simulink library "PowerFlowLib"  (Simulink 8.1)
settings: Solver=ode45  StartTime=0.0  StopTime=10.0  RelTol=1e-3
undefined symbols (not defined in the file or in its folder): AirProp, C, F1, Fanmap, Fld1, Fld2, Fluid, fueltankdata, HydProp, HydraulicLoad, IBFD_exc, L, LoadFluidProps, magnitude, MSSN, n_alghts, PumpProp, pwr_alghts, R_fd_exc, Rcore, Ts, VBFD_exc
libraries: PowerFlowLib x33, simulink x15, powerlib_extras x2, dspstat3 x2
(part 6 of 11)

== system PowerFlowLib/Energy & Power Systems/Thermal/Fuel & Oil ==
  Cold Plate : Subsystem  mask{fld=Fuel, Tw_init=50, C_wall=60000, H0=10000, A=0.033217, mdot0=2, Q0=12750, Tw0=50, Tin0=10}
      mask prompts: fld "Fluid Type"; Tw_init "Initial Wall Temperature [°C]"; C_wall "Wall Heat Capacitance [J/K]"; H0 "Heat Transfer Coefficient [W/m²K]"; A "Heat Transfer Area [m²]"; mdot0 "Mass Flow Rate [kg/s]"; Q0 "Heat Absorption Rate [W]"; Tw0 "Wall Temperature [°C]"; Tin0 "Fluid Inlet Temperature [°C]"
      mask init:
      | load Fluids
      | eval(['Fluid = Fluid.',get_param(gcb,'fld'),';']);
      | 
      | 
      | area = -(mdot0*Fluid.cp/H0)*...
      |               log(1-Q0/(mdot0*Fluid.cp*(Tw0-Tin0)));
      |           
      |           
      | set_param(gcb,'A',num2str(area));
      mask TypeOptions fld: Fuel | Water
      mask Display:
      | text(0.5,0.95,['{\bf ',fld,' Cold Plate}'],'TexMode','on','horizontalAlignment', 'center')
      | 
      | port_label('input',1,'Heat Load [W]')
      | port_label('input',2,'Flow In')
      | port_label('output',1,'Flow Out')
  Flow Junction : Subsystem  Description=TwoPhase  mask{fld=Fuel, V=.05, Bm=10^5, initPres=6000, initTemp=30}
      mask prompts: fld "Fluid Type"; V "Volume (m^3)"; Bm "Bulk Modulus (kPa)"; initPres "Initial Pressure (kPa)"; initTemp "Initial Temperature (C)"
      mask init:
      | initTemp = initTemp + 273.15;
      | if strcmp(get_param(gcb,'fld'),'Fuel') == 1
      |     load FluidProp_JetA3638
      |     eval(['F1 = FuelProp;']);
      | elseif strcmp(get_param(gcb,'fld'),'Oil') == 1
      |     load OilProp
      |     eval(['F1 = OilProp;']);
      | else
      |     error(['Incorrect fluid chosen in block: ',gcb,'.  Check initialization commands.'])
      | end
      mask TypeOptions fld: Fuel | Oil
      mask Display:
      | image(imread('MergeImage.png'))
      | 
      | port_label('input',1,'{\bf mdot Out}','TexMode','on')
      | port_label('input',2,'{\bf Flow 1}','TexMode','on')
      | port_label('input',3,'{\bf Flow 2}','TexMode','on')
      | port_label('input',4,'{\bf Flow 3}','TexMode','on')
      | 
      | port_label('output',1,'{\bfFlow }','TexMode','on')
  Fluid Pump : Subsystem  mask(Pump){fld=Fuel, maptype=Pressure (kPa) vs. Vol. Flow Rate (m³/hr), map=B737_mech_fuel1, map_load=off, SG=0.82, pump_eff=.75, heat_out=on, AC_pwr=on, pf=1, mech_pwr=off}
      mask prompts: fld "Fluid Type"; maptype "Map Type"; map "Select Map"; map_load "Load new map?"; SG "Specific Gravity of Flow"; pump_eff "Pump Overall Efficiency"; heat_out "Add heat to flow?"; AC_pwr "AC Powered?"; pf "Power Factor"; mech_pwr "Mechanically Driven?"
      mask help:
      | Input 1: Input Flow Bus
      | Input 2: Shaft RPM (rpm)
      | Input 3: Upstream Pressure (kPa)
      |
      | Output 1: Output Flow Bus
      | Output 2: Pump Power Bus (mech or elec)
      | Optional: Pump Heat Generated (kW)
      mask init:
      | if exist('PumpProp') == 0
      |   load('PumpProp.mat')
      | end
      | h      = get_param(gcb,'handle');   % Get block handle
      | blk    = gcb; 
      | hblock = get(h);     % Parse out handles structure
      | 
      | if strcmp(get_param(gcb,'fld'),'Fuel') == 1
      |     load FluidProp_JetA3638
      |     eval(['F1 = FuelProp;']);
      | elseif strcmp(get_param(gcb,'fld'),'Oil') == 1
      |     load OilProp
      |     eval(['F1 = OilProp;']);
      | else
      |     error(['Incorrect fluid chosen in block: ',gcb,'.  Check initialization commands.'])
      | end
      | 
      | if strcmp(hblock.maptype,'Head (m) vs. Vol. Flow Rate (m³/hr)') == 1;
      |     set_param([blk,'/switchcase'],'Value','1');
      |     set_param([blk,'/Pump Vol. FlowRate'],'Table',['PumpProp.',map,'.q']);
      |     set_param([blk,'/Pump Vol. FlowRate'],'BreakpointsForDimension1',['PumpProp.',map,'.head']);
      | elseif strcmp(hblock.maptype,'Pressure (kPa) vs. Vol. Flow Rate (m³/hr)') == 1;
      |     set_param([blk,'/switchcase'],'Value','2');
      |     set_param([blk,'/Pump Vol. FlowRate'],'Table',['PumpProp.',map,'.q']);
      |     set_param([blk,'/Pump Vol. FlowRate'],'BreakpointsForDimension1',['PumpProp.',map,'.pres']);
      | elseif strcmp(hblock.maptype,'Pressure (bar) vs. Vol. Flow Rate (m³/hr)') == 1;
      |     set_param([blk,'/switchcase'],'Value','3');
      |     set_param([blk,'/Pump Vol. FlowRate'],'Table',['PumpProp.',map,'.q']);
      |     set_param([blk,'/Pump Vol. FlowRate'],'BreakpointsForDimension1',['PumpProp.',map,'.pres']);
      | else
      |     error('see pump mask callback for map type');
      | end    
      | 
      | % TURNING ON/OFF PUMP HEAT GENERATION OUTPUT
      | if strcmp(hblock.heat_out,'on') == 1;   % adding heat to fluid flow
      |     set_param([blk,'/heat_switch'],'Gain','1')  % turn on heat added to flow
      |     try
      |         delete_block([blk,'/Heat (kW)'])
      |     catch
      |     end
      |     delete_unconnected_lines(blk)
      |         
      | elseif strcmp(hblock.heat_out,'off') == 1; % not adding heat to fluid flow
      |     set_param([blk,'/heat_switch'],'Gain','0')  % adding no heat to flow
      |     try
      |         add_block('built-in/Outport',[blk,'/Heat (kW)'],'Position',[800 200 830 214]);
      |         add_line(blk,'W to kW/1','Heat (kW)/1')
      |     catch
      |     end
      | end
      | 
      | clear h blk hblock
      settings: OpenFcn=|
      | if exist('PumpProp') == 0
      |   load('PumpProp.mat')
      | end
      | open_system(gcb,'mask')
      mask TypeOptions fld: Fuel | Oil
      mask TypeOptions maptype: Head (m) vs. Vol. Flow Rate (m³/hr) | Pressure (kPa) vs. Vol. Flow Rate (m³/hr) | Pressure (bar) vs. Vol. Flow Rate (m³/hr)
      mask Callback maptype:
      | h      = get_param(gcb,'handle');   % Get block handle
      | blk    = gcb;
      | hblock = get(h);     % Parse out handles structure
      | 
      | if strcmp(hblock.maptype,'Head (m) vs. Vol. Flow Rate (m³/hr)') == 1;
      |     set_param([blk,'/switchcase'],'Value','1');
      |     set_param([blk,'/Pump Vol. FlowRate'],'Table',['PumpProp.',hblock.map,'.q']);
      |     set_param([blk,'/Pump Vol. FlowRate'],'BreakpointsForDimension1',['PumpProp.',hblock.map,'.head']);
      | elseif strcmp(hblock.maptype,'Pressure (kPa) vs. Vol. Flow Rate (m³/hr)') == 1;
      |     set_param([blk,'/switchcase'],'Value','2');
      |     set_param([blk,'/Pump Vol. FlowRate'],'Table',['PumpProp.',hblock.map,'.q']);
      |     set_param([blk,'/Pump Vol. FlowRate'],'BreakpointsForDimension1',['PumpProp.',hblock.map,'.pres']);
      | elseif strcmp(hblock.maptype,'Pressure (bar) vs. Vol. Flow Rate (m³/hr)') == 1;
      |     set_param([blk,'/switchcase'],'Value','3');
      |     set_param([blk,'/Pump Vol. FlowRate'],'Table',['PumpProp.',hblock.map,'.q']);
      |     set_param([blk,'/Pump Vol. FlowRate'],'BreakpointsForDimension1',['PumpProp.',hblock.map,'.pres']);
      | else
      |     error('see pump mask callback for map type');
      | end
      | 
      | clear h blk hblock
      mask TypeOptions map: B737_mech_fuel1 | B737_mech_fuel2 | B737_mech_fuel3 | B737_AC_fuel1 | B737_AC_oil1
      mask Callback map:
      | h      = get_param(gcb,'handle');   % Get block handle
      | blk    = gcb;
      | hblock = get(h);     % Parse out handles structure
      | vals = get_param(blk,'MaskValues');
      | % find all installed pumps in the PumpProp.mat file
      | pumps = fieldnames(PumpProp);
      | indx = strfind(pumps, 'units');
      | indx = find(not(cellfun('isempty', indx)));
      | pumps(indx) = [];      % removing the units entry
      | 
      | for i = 1:size(pumps,1);
      |    if i==1;
      |     pmpstr = pumps{i};
      |    else
      |        pmpstr = strcat(pmpstr,char(124),pumps{i});
      |    end
      | end
      | 
      | % Get the mask parameter values. This is a cell array of strings.
      | styl = get_param(blk,'MaskStyles');
      | 
      | vis = get_param(blk,'MaskVisibilities');
      | str = get_param(blk,'MaskPromptString');
      | 
      | % fill the mask with the parameters
      | set_param(blk,'MaskVisibilities',vis,'MaskPromptString',str,'MaskValues',vals,'MaskStyles',[styl(1:2);strcat('popup(',pmpstr,')');styl(4:10)]);
      | 
      | clear h blk hblock styl vals vis str pmpstr i indx pumps
      mask Callback AC_pwr:
      | h      = get_param(gcb,'handle');   % Get block handle
      | blk    = gcb;
      | hblock = get(h);     % Parse out handles structure
      | 
      | vis = get_param(blk,'MaskVisibilities');
      | 
      | if strcmp(hblock.AC_pwr,'off') == 1;
      |     % fill the mask with the parameters
      |     set_param(blk,'MaskVisibilities',[vis(1:8);'off';vis(10)])
      |     set_param(blk,'mech_pwr','on');
      |     set_param([blk,'/pwr_switch'],'Value','0.5')
      | elseif strcmp(hblock.AC_pwr,'on') == 1;
      |     % fill the mask with the parameters
      |     set_param(blk,'MaskVisibilities',[vis(1:8);'on';vis(10)])
      |     set_param(blk,'mech_pwr','off');
      |     set_param([blk,'/pwr_switch'],'Value','0')
      | end
      | 
      | clear h blk hblock vis
      mask Callback mech_pwr:
      | h      = get_param(gcb,'handle');   % Get block handle
      | blk    = gcb;
      | hblock = get(h);     % Parse out handles structure
      | 
      | vis = get_param(blk,'MaskVisibilities');
      | 
      | if strcmp(hblock.mech_pwr,'off') == 1;
      |     % fill the mask with the parameters
      |     set_param(blk,'MaskVisibilities',[vis(1:8);'on';vis(10)])
      |     set_param(blk,'AC_pwr','on');
      |     set_param([blk,'/pwr_switch'],'Value','0')
      | elseif strcmp(hblock.mech_pwr,'on') == 1;
      |     % fill the mask with the parameters
      |     set_param(blk,'MaskVisibilities',[vis(1:8);'off';vis(10)])
      |     set_param(blk,'AC_pwr','off');
      |     set_param([blk,'/pwr_switch'],'Value','0.5')
      | end
      | clear h blk hblock vis
      mask Display:
      | image(imread('pump.png'));
      | 
      | port_label('input',1,'{\bf Flow In}','TexMode','on')
      | port_label('input',2,'{\bf w (rpm)}','TexMode','on')
      | port_label('input',3,'{\bf P_o_u_t (kPa)}','TexMode','on')
      | 
      | port_label('output',1,'{\bf Flow Out}','TexMode','on')
      | port_label('output',2,'{\bf Pump Power}','TexMode','on')
      | 
      | h      = get_param(gcb,'handle');   % Get block handle
      | hblock = get(h);     % Parse out handles structure
      | 
      | if heat_out == 0
      |     port_label('output',3,'{\bf Pump Heat [kW]}','TexMode','on')
      | end
  Fluid Tank : Subsystem  mask(Fluid Tank){fld=Fuel, fileslct=off, filename=fueltank_area.m, filedir=fueltank_area.m, tank_loc=Left Wing Tank, areaprompt2=off, max_vol=3.2, m_init=2500, fld_Tint=0, ull_Tint=30, Pover=100, HTC_fg=14.2, wallHXF=off, wetHTC=14.2, dryHTC=14.2, Qinternal=0}
      mask prompts: fld "Fluid Type"; fileslct "Browse for area .m file?"; filename "Fuel Tank Area .m File"; filedir "Area .m File Directory"; tank_loc "Select Tank"; areaprompt2 "Edit Fuel Tank Area Manually?"; max_vol "Maximum Tank Volume [m³]"; m_init "Initial Fluid Mass [kg]"; fld_Tint "Initial Fluid Temperature [°C]"; ull_Tint "Initial Ullage Temperature [°C]"; Pover "Tank Pressurization [kPa]"; HTC_fg "Liquid to Ullage HTC [W/m² K]"; wallHXF "Enable Wall Heat Transfer"; wetHTC "Wall to Liquid HTC [W/m² K]"; dryHTC "Wall to Ullage HTC [W/m² K]"; Qinternal "Internal Heat Load [W]"
      mask help:
      | Input 1: Input Flow Bus
      | Input 2: Flow Rate Out [kg/s]
      | Input 3: Ambient Pressure [kPa]
      | Input 4: Heat Load [W]
      | Input 5: Initial Wall Temps. Vector [K]
      |
      | Output 1: Output Flow Bus
      | Output 2: Tank mass [kg]
      | Output 3: Ullage Temp. [K]
      mask init:
      | h      = get_param(gcb,'handle');   % Get block handle
      | blk    = gcb; 
      | hblock = get(h);     % Parse out handles structure 
      | 
      | if strcmp(get_param(gcb,'fld'),'Fuel') == 1
      |     load FluidProp_JetA3638
      |     eval(['F1 = FuelProp;']);
      | elseif strcmp(get_param(gcb,'fld'),'Oil') == 1
      |     load OilProp
      |     eval(['F1 = OilProp;']);
      | else
      |     error(['Incorrect fluid chosen in block: ',gcb,'.  Check initialization commands.'])
      | end
      | 
      | if exist('AirProp') == 0
      |     load AirProp.mat
      | end
      | %{
      | % the following checks for the existance of a file and loads the
      | % spreadsheet into variables that populate the 2D lookup table
      | 
      | if isempty(filedir) == 0;
      |     areadata = xlsread(filedir,1);
      |     vol_per = areadata(:,1);
      |     wall_area = [areadata(:,2:size(areadata,2))];
      | end
      | %}
      | if strcmp(hblock.areaprompt2,'on') == 0;
      |     
      |     % run the selected fuel area file
      |     if ~isempty(strfind(filename,'.m'))
      |         try
      |             run(filename(1:strfind(filename,'.m')-1))       % removing the .m extension and loading the file
      |         catch
      |             error(['Unable to load selected fuel area file in ',blk,'. Verify the file is a .m script file and on the MATLAB Path'])
      |         end
      |     else
      |         try
      |             run(filename)
      |         catch
      |             error(['Unable to load selected fuel area file in ',blk,'. Verify the file is a .m script file and on the MATLAB Path'])
      |         end
      |     end
      |    
      |     switch hblock.tank_loc
      |         case 'Left Wing Tank'
      |             set_param([blk,'/Wall Heat Transfer/volume_%'],'Table', 'fueltankdata.leftwingtank');
      |             %BP1values = strcat('[',num2str(linspace(0,1,size(fueltankdata.leftwingtank,1))),']');
      |             %BP2values = strcat('[',num2str(linspace(1,size(fueltankdata.leftwingtank,2),size(fueltankdata.leftwingtank,2))),']');
      |             set_param([blk,'/Wall Heat Transfer/volume_%'],'BreakpointsForDimension1', 'linspace(0,1,11)');
      |             set_param([blk,'/Wall Heat Transfer/volume_%'],'BreakpointsForDimension2', 'linspace(1,6,6)');
      |             set_param([blk,'/Wall Heat Transfer/Walls 1 to n'],'Value','1:size(fueltankdata.leftwingtank,2)');
      |             set_param([blk,'/Wall Heat Transfer/total area'],'Bias','-[fueltankdata.leftwingtank(11,:)]');
      |             set_param([blk,'/ullage-fluid_area'],'Value','fueltankdata.leftwingtank(2,2)');
      |             
      |         case 'Center Tank'
      |             set_param([blk,'/Wall Heat Transfer/volume_%'],'Table', 'fueltankdata.centertank');
      |             %BP1values = strcat('[',num2str(linspace(0,1,size(fueltankdata.centertank,1))),']');
      |             %BP2values = strcat('[',num2str(linspace(1,size(fueltankdata.centertank,2),size(fueltankdata.centertank,2))),']');
      |             set_param([blk,'/Wall Heat Transfer/volume_%'],'BreakpointsForDimension1', 'linspace(0,1,11)');
      |             set_param([blk,'/Wall Heat Transfer/volume_%'],'BreakpointsForDimension2', 'linspace(1,6,6)');
      |             set_param([blk,'/Wall Heat Transfer/Walls 1 to n'],'Value','1:size(fueltankdata.centertank,2)');
      |             set_param([blk,'/Wall Heat Transfer/total area'],'Bias','-[fueltankdata.centertank(11,:)]');
      |             set_param([blk,'/ullage-fluid_area'],'Value','fueltankdata.centertank(2,2)');
      |             
      |         case 'Right Wing Tank'
      |             set_param([blk,'/Wall Heat Transfer/volume_%'],'Table', 'fueltankdata.rightwingtank');
      |             %BP1values = strcat('[',num2str(linspace(0,1,size(fueltankdata.rightwingtank,1))),']');
      |             %BP2values = strcat('[',num2str(linspace(1,size(fueltankdata.rightwingtank,2),size(fueltankdata.rightwingtank,2))),']');
      |             set_param([blk,'/Wall Heat Transfer/volume_%'],'BreakpointsForDimension1', 'linspace(0,1,11)');
      |             set_param([blk,'/Wall Heat Transfer/volume_%'],'BreakpointsForDimension2', 'linspace(1,6,6)');
      |             set_param([blk,'/Wall Heat Transfer/Walls 1 to n'],'Value','1:size(fueltankdata.rightwingtank,2)');
      |             set_param([blk,'/Wall Heat Transfer/total area'],'Bias','-[fueltankdata.rightwingtank(11,:)]');
      |             set_param([blk,'/ullage-fluid_area'],'Value','fueltankdata.rightwingtank(2,2)');
      |             
      |     end
      |     
      | end
      | 
      | %% CHECK FOR VOLUME OF FUEL BEING GREATER THAN VOLUME OF TANK
      | X = F1.P;
      | Y = F1.T;
      | delx = X(2)-X(1);
      | dely = Y(2)-Y(1);
      | xref = round((Pover + 101 - X(1))/delx);
      | yref = round((fld_Tint + 273 - Y(1))/dely);
      | 
      | rhoIC = F1.Rho_pt(xref,yref);
      | volIC = m_init / rhoIC;
      | 
      | if volIC > max_vol
      |     error('Initial volume of fluid is greater than max volume of tank.')
      | end
      | 
      | 
      | clear h blk hblock
      mask TypeOptions fld: Fuel | Oil
      mask Callback fileslct:
      | h      = get_param(gcb,'handle');   % Get block handle
      | blk    = gcb;
      | hblock = get(h);     % Parse out handles structure
      | 
      | if strcmp(hblock.fileslct,'on') == 1;
      |     set_param(gcb,'areaprompt2','off');     % turn off manual switch
      |     RR_SetPerfSlct(2,0);                    % call uiopen script
      |     set_param(gcb,'fileslct','off')
      | end
      | 
      | clear h blk hblock
      mask TypeOptions tank_loc: Left Wing Tank | Center Tank | Right Wing Tank
      mask Callback areaprompt2:
      | h      = get_param(gcb,'handle');   % Get block handle
      | blk    = gcb;
      | hblock = get(h);     % Parse out handles structure
      | 
      | if strcmp(hblock.areaprompt2,'on') == 1;
      |     set_param(gcb,'fileslct','off');
      |     open_system([blk, '/Wall Heat Transfer/volume_%']);
      | end
      mask Callback wallHXF:
      | h      = get_param(gcb,'handle');   % Get block handle
      | blk    = gcb;
      | hblock = get(h);     % Parse out handles structure
      | 
      | if strcmp(hblock.wallHXF,'on') == 1;
      |     set_param([blk,'/enable_wall_HXF'],'Value','1');
      | else
      |     set_param([blk,'/enable_wall_HXF'],'Value','0');
      | end
      | 
      | clear h blk hblock
      mask Display:
      | image(imread('fueltank.jpg'))
      | 
      | port_label('input',1,'{\bf Flow In}','TexMode','on')
      | port_label('input',2,'{\bf Flow Rate Out}','TexMode','on')
      | port_label('input',3,'{\bf P_a_m_b [kPa]}','TexMode','on')
      | port_label('input',4,'{\bf Heat Load [kW]}','TexMode','on')
      | port_label('input',5,'{\bf Wall Temp. [K]}','TexMode','on')
      | 
      | port_label('output',1,'{\bf Flow Out }','TexMode','on')
      | port_label('output',2,'{\bf Fluid Mass [kg]}','TexMode','on')
      | port_label('output',3,'{\bf Ullage Temp. [K]}','TexMode','on')
  Fuel Control : Subsystem  mask(Fuel Control){}
      mask help: Manages fuel bypass and fuel sent to the engine.
      mask Display:
      | port_label('input',1,'{\bf Fuel Need}','TexMode','on')
      | port_label('input',2,'{\bf Fuel In}','TexMode','on')
      | 
      | 
      | port_label('output',1,'{\bf Fuel to Eng.}','TexMode','on')
      | port_label('output',2,'{\bf Fuel Return}','TexMode','on')
  Heat Exchanger : Subsystem  mask(Single-phase Fluid Heat Exchanger){fld1=Fuel, fld2=Air, Tw_init=0, C_wall=60000, Tw0=30, Q0=20000, H1_0=10000, A1=0.11584, mdot1_0=2, Tin1_0=10, Pin1_0=100, H2_0=10000, A2=0.13814, mdot2_0=2, Tin2_0=50, Pin2_0=100}
      mask prompts: fld1 "Fluid Type 1"; fld2 "Fluid Type 2"; Tw_init "Initial Wall Temperature [°C]"; C_wall "Wall Heat Capacitance  [J/K]"; Tw0 "Wall Temperature [°C]"; Q0 "Heat Transfer Rate [W]"; H1_0 "Heat Transfer Coefficient [W/m²K]"; A1 "Heat Transfer Area [m²]"; mdot1_0 "Mass Flow Rate [kg/s]"; Tin1_0 "Fluid Inlet Temperature [°C]"; Pin1_0 "Fluid Inlet Pressure [kPa]"; H2_0 "Heat Transfer Coefficient [W/m²K]"; A2 "Heat Transfer Area [m²]"; mdot2_0 "Mass Flow Rate [kg/s]"; Tin2_0 "Fluid Inlet Temperature [°C]"; Pin2_0 "Fluid Inlet Pressure [kPa]"
      mask help: Tracks the time rate of change of the wall temperature and exit flow temperatures.
      mask init:
      | % the following if statements look at the selected fluid for the primary
      | % and secondary flow. based upon this selection, the appropriate fluid
      | % property file is loaded and saved locally as Fld1 or Fld2
      | % If an incorrect selection is made, then an error is displayed. This would
      | % occur if a user adds a new fluid selection without updating this
      | % initialization code
      | if strcmp(get_param(gcb,'fld1'),'Air') == 1
      |     load AirProp
      |     eval(['Fld1 = AirProp;']);
      | elseif strcmp(get_param(gcb,'fld1'),'Fuel') == 1
      |     load FluidProp_JetA3638
      |     eval(['Fld1 = FuelProp;']);
      | elseif strcmp(get_param(gcb,'fld1'),'Oil') == 1
      |     load OilProp
      |     eval(['Fld1 = OilProp;']);
      | elseif strcmp(get_param(gcb,'fld1'),'PAO') == 1
      |     load PAOProp
      |     eval(['Fld1 = PAOProp;']);
      | else
      |     error(['Incorrect fluid chosen in block: ',gcb,'.  Check initialization commands.'])
      | end
      | 
      | if strcmp(get_param(gcb,'fld2'),'Air') == 1 
      |     load AirProp
      |     eval(['Fld2 = AirProp;']);
      | elseif strcmp(get_param(gcb,'fld2'),'Fuel') == 1
      |     load FluidProp_JetA3638
      |     eval(['Fld2 = FuelProp;']);
      | elseif strcmp(get_param(gcb,'fld2'),'Oil') == 1
      |     load OilProp
      |     eval(['Fld2 = OilProp;']);
      | elseif strcmp(get_param(gcb,'fld2'),'PAO') == 1
      |     load PAOProp
      |     eval(['Fld2 = PAOProp;']);
      | else
      |     error(['Incorrect fluid chosen in block: ',gcb,'.  Check initialization commands.'])
      | end
      | 
      | % determining the location of Cp in the look up table, based upon mask
      | % parameters
      | X = Fld1.P;
      | Y = Fld1.T;
      | delx = X(2)-X(1);
      | dely = Y(2)-Y(1);
      | xref = max(round((Pin1_0 - X(1))/delx),1);
      | 
      | % OilProp has a 1D table for Cp --> xref = 1
      | if strcmp(get_param(gcb,'fld1'),'Oil') == 1; xref = 1; end;
      | yref = round((Tin1_0 + 273 - Y(1))/dely);
      | 
      | % heat exchanger area required to achieve the nominal values defined in the
      | % GUI -- based upon log temperature difference relationships
      | area1 = -(mdot1_0*Fld1.Cp_pt(xref,yref)*1000/H1_0)*...
      |               log(1-Q0/(mdot1_0*Fld1.Cp_pt(xref,yref)*1000*abs(Tw0-Tin1_0)));
      | set_param(gcb,'A1',num2str(area1));          
      | 
      | % the following code is identical to the previous block, but is for Fld2
      | X = Fld2.P;
      | Y = Fld2.T;
      | delx = X(2)-X(1);
      | dely = Y(2)-Y(1);
      | xref = max(round((Pin2_0 - X(1))/delx),1);
      | if strcmp(get_param(gcb,'fld2'),'Oil') == 1; xref = 1; end;
      | yref = round((Tin2_0 + 273 - Y(1))/dely);
      | 
      | area2 = -(mdot2_0*Fld2.Cp_pt(xref,yref)*1000/H2_0)*...
      |               log(1-Q0/(mdot2_0*Fld2.Cp_pt(xref,yref)*1000*abs(-Tw0+Tin2_0)));   
      | set_param(gcb,'A2',num2str(area2));
      mask TypeOptions fld1: Fuel | Air | Oil | PAO
      mask TypeOptions fld2: Fuel | Air | Oil | PAO
      mask Display:
      | text(0.5,0.95,['{\bf ',fld1,'/',fld2,' HX}'],'TexMode','on','horizontalAlignment', 'center')
      | 
      | port_label('input',1,[fld1,' In'])
      | port_label('input',2,[fld2,' In'])
      | port_label('output',1,[fld1,' Out'])
      | port_label('output',2,[fld2,' Out'])
  Stochastic Heat Loads : Subsystem  mask(Heat Loads){noise_pwr=.5, samp_time=10, seed=23341}
      mask prompts: noise_pwr "Noise Power"; samp_time "Sample Time"
      mask help:
      | Increase the flow temperature using nomally distributed white noise.  Noise power and sample time affect the magnitude of the temperature increase.  Use a fixed seed for repeatable heat loads.
      |
      | Temp. Out = Temp. In + Integral(white noise)
      |
      | Integration has a lower saturation of zero.
      mask Display:
      | port_label('output',1,'{\bf Flow Out}','TexMode','on')
      | port_label('input',1,'{\bf Flow In}','TexMode','on')

== system PowerFlowLib/Energy & Power Systems/Electrical/Battery/BATTERY ==
  note: BUS VOLTAGE SYNTHESIS
      | SERIES CONNECTION
  note: TERMINAL VOLTAGE
      | AND LOSS CALC
      |  AT EACH CELL
  note: STATE OF CHARGE
      | DETERMINATION
  note: OUT SIGNAL DEFINITIONS
      |
      | 1 - DISCHARGE
      | 2 - CHARGE
      | 3 - OPEN CIRCUIT
  CT OUT : Inport
  CT IN : Inport  Port=2
  BUS VOLTAGE : Subsystem
  Bus Creator : BusCreator  Inputs=2
  Constant : Constant  Value=NO_CELLS
  Constant3 : Constant  Value=INITIAL_SOC
  Constant4 : Constant  Value=NO_MODULES
  NET  CHARGE/DISCHARGE DETECTION : Subsystem
  SINGLE CELL VOLT OUT : Subsystem
  "SOC " : Subsystem
  data_sink : PowerFlowLib/Support Functions//Tools/data_sink
  VDC : Outport
  PLOSS : Outport  Port=2
  wires:
  NET  CHARGE/DISCHARGE DETECTION/3(CHG CURRENT) -> SINGLE CELL VOLT OUT/3(CHG CT), "SOC "/3(CHG CT)
  NET  CHARGE/DISCHARGE DETECTION/2(DCHG CURRENT) -> SINGLE CELL VOLT OUT/2(DCHG CT), "SOC "/2(DCHG CT)
  BUS VOLTAGE/2(BATTERY_ PLOSS) -> PLOSS/1
  Constant4/1 -> NET  CHARGE/DISCHARGE DETECTION/3(NO_MODULES)
  BUS VOLTAGE/1(BUS VOLTAGE) -> VDC/1, Bus Creator/1  "VDC (V)"
  Constant/1 -> BUS VOLTAGE/2(NO_CELLS)
  SINGLE CELL VOLT OUT/2(POWER LOSS) -> BUS VOLTAGE/3(PLOSS/CELL)
  SINGLE CELL VOLT OUT/1(CELL VOLT) -> BUS VOLTAGE/1(VOLT/CELL)
  Constant3/1 -> "SOC "/1(INITIAL SOC)
  "SOC "/1(DYNAMIC SOC) -> SINGLE CELL VOLT OUT/4(SOC)
  NET  CHARGE/DISCHARGE DETECTION/1(CHG/DCHG SIGNAL) -> SINGLE CELL VOLT OUT/1(CHG_DCHG_SIGNAL), "SOC "/4(CHG_DCHG_SIGNAL)
  CT OUT/1 -> NET  CHARGE/DISCHARGE DETECTION/1(CT OUT)
  CT IN/1 -> NET  CHARGE/DISCHARGE DETECTION/2(CT IN)
  Bus Creator/1 -> data_sink/1
  "SOC "/2(NET DCHG CURRENT) -> Bus Creator/2  "Net Dchg Current (A)"

== system PowerFlowLib/Energy & Power Systems/Electrical/Converters/Boost converter (CCM only; ideal averaged) ==
  vin : Inport
  iout : Inport  Port=2
  d(t) : Inport  Port=3
  1/C : Gain  Gain=1/C  SaturateOnIntegerOverflow=on  OutDataTypeStr=Inherit: Same as input  ParamDataTypeStr=Inherit: Same as input
  1/L : Gain  Gain=1/L  SaturateOnIntegerOverflow=on  OutDataTypeStr=Inherit: Same as input  ParamDataTypeStr=Inherit: Same as input
  Dot Product : DotProduct  InputSameDT=on  OutDataTypeStr=Inherit: Inherit via internal rule
  Dot Product2 : DotProduct  InputSameDT=on  OutDataTypeStr=Inherit: Inherit via internal rule
  Fcn : Fcn  Expr=1-u
  Sum : Sum  Inputs=+-  SaturateOnIntegerOverflow=on  InputSameDT=on  OutDataTypeStr=Inherit: Same as first input
  Sum1 : Sum  Inputs=+-  SaturateOnIntegerOverflow=on  InputSameDT=on  OutDataTypeStr=Inherit: Same as first input
  iL : Integrator  LimitOutput=on  LowerSaturationLimit=0
  vc : Integrator
  vout : Outport
  iin : Outport  Port=2
  q : Outport  Port=3
  wires:
  iL/1 -> iin/1, Dot Product2/1
  vc/1 -> Dot Product/2, vout/1
  iout/1 -> Sum1/2
  Sum1/1 -> 1/C/1
  1/C/1 -> vc/1
  Dot Product2/1 -> Sum1/1
  Fcn/1 -> Dot Product2/2, Dot Product/1
  vin/1 -> Sum/1
  Dot Product/1 -> Sum/2
  Sum/1 -> 1/L/1
  1/L/1 -> iL/1
  d(t)/1 -> Fcn/1, q/1

== system PowerFlowLib/Energy & Power Systems/Electrical/Converters/Buck converter (CCM only; ideal averaged) ==
  vin : Inport
  iout : Inport  Port=2
  d(t) : Inport  Port=3
  1/C : Gain  Gain=1/C  SaturateOnIntegerOverflow=on  OutDataTypeStr=Inherit: Same as input  ParamDataTypeStr=Inherit: Same as input
  1/L : Gain  Gain=1/L  SaturateOnIntegerOverflow=on  OutDataTypeStr=Inherit: Same as input  ParamDataTypeStr=Inherit: Same as input
  Dot Product : DotProduct  InputSameDT=on  OutDataTypeStr=Inherit: Inherit via internal rule
  Dot Product1 : DotProduct  InputSameDT=on  OutDataTypeStr=Inherit: Inherit via internal rule
  Sum : Sum  Inputs=+-  SaturateOnIntegerOverflow=on  InputSameDT=on  OutDataTypeStr=Inherit: Same as first input
  Sum1 : Sum  Inputs=+-  SaturateOnIntegerOverflow=on  InputSameDT=on  OutDataTypeStr=Inherit: Same as first input
  iLstate : Integrator  LimitOutput=on  LowerSaturationLimit=0
  vc : Integrator  LowerSaturationLimit=0
  vout : Outport
  iL : Outport  Port=2
  iin : Outport  Port=3
  q : Outport  Port=4
  wires:
  Dot Product1/1 -> iin/1
  iLstate/1 -> Dot Product1/1, Sum1/1, iL/1
  vc/1 -> Sum/2, vout/1
  1/C/1 -> vc/1
  Sum1/1 -> 1/C/1
  iout/1 -> Sum1/2
  vin/1 -> Dot Product/1
  Dot Product/1 -> Sum/1
  1/L/1 -> iLstate/1
  Sum/1 -> 1/L/1
  d(t)/1 -> q/1, Dot Product1/2, Dot Product/2

== system PowerFlowLib/Energy & Power Systems/Electrical/Converters/Buck-boost converter   (CCM only; ideal averaged) ==
  vin : Inport
  iout : Inport  Port=2
  d(t) : Inport  Port=3
  1/C : Gain  Gain=1/C  SaturateOnIntegerOverflow=on  OutDataTypeStr=Inherit: Same as input  ParamDataTypeStr=Inherit: Same as input
  1/L : Gain  Gain=1/L  SaturateOnIntegerOverflow=on  OutDataTypeStr=Inherit: Same as input  ParamDataTypeStr=Inherit: Same as input
  Dot Product{,2..4} (4 alike) : DotProduct  InputSameDT=on  OutDataTypeStr=Inherit: Inherit via internal rule
  Fcn : Fcn  Expr=1-u
  Sum : Sum  SaturateOnIntegerOverflow=on  InputSameDT=on  OutDataTypeStr=Inherit: Same as first input
  Sum1 : Sum  Inputs=--  SaturateOnIntegerOverflow=on  InputSameDT=on  OutDataTypeStr=Inherit: Same as first input
  iL : Integrator
  vc : Integrator
  vout : Outport
  iin : Outport  Port=2
  q : Outport  Port=3
  wires:
  iL/1 -> Dot Product4/1, Dot Product3/1
  Dot Product4/1 -> iin/1
  vc/1 -> Dot Product2/2, vout/1
  Fcn/1 -> Dot Product3/2, Dot Product2/1
  Dot Product3/1 -> Sum1/1
  Dot Product2/1 -> Sum/2
  vin/1 -> Dot Product/1
  Dot Product/1 -> Sum/1
  1/L/1 -> iL/1
  Sum/1 -> 1/L/1
  1/C/1 -> vc/1
  Sum1/1 -> 1/C/1
  iout/1 -> Sum1/2
  d(t)/1 -> Dot Product4/2, Dot Product/2, q/1, Fcn/1

== system PowerFlowLib/Energy & Power Systems/Electrical/Converters/Chopper (Averaged) ==
  vin : Inport
  iout : Inport  Port=2
  d(t) : Inport  Port=3
  Dot Product : DotProduct  InputSameDT=on  OutDataTypeStr=Inherit: Inherit via internal rule
  Dot Product1 : DotProduct  InputSameDT=on  OutDataTypeStr=Inherit: Inherit via internal rule
  Terminator : Terminator
  duty ratio : Subsystem
  vout : Outport
  iin : Outport  Port=2
  q : Outport  Port=3
  wires:
  Dot Product1/1 -> iin/1
  duty ratio/1(d1(t)) -> q/1, Dot Product1/2, Dot Product/2
  vin/1 -> Dot Product/1
  duty ratio/2(d2(t)) -> Terminator/1
  d(t)/1 -> duty ratio/1(d(t))
  Dot Product/1 -> vout/1
  iout/1 -> Dot Product1/1

== system PowerFlowLib/Energy & Power Systems/Electrical/Converters/Chopper (Averaged)1 ==
  vin : Inport
  q : Inport  Port=2
  1/R : Gain  Gain=1/(R_fd_exc*VBFD_exc/IBFD_exc)/100/2*3/100  SaturateOnIntegerOverflow=on  OutDataTypeStr=Inherit: Same as input  ParamDataTypeStr=Inherit: Same as input
  Dot Product : DotProduct  InputSameDT=on  OutDataTypeStr=Inherit: Inherit via internal rule
  Dot Product1 : DotProduct  InputSameDT=on  OutDataTypeStr=Inherit: Inherit via internal rule
  Gain2 : Gain  Gain=1000*2/3
  Saturation : Saturate  UpperLimit=1  LowerLimit=0
  iout : Outport
  iin : Outport  Port=2
  wires:
  Gain2/1 -> iout/1, Dot Product1/1
  vin/1 -> Dot Product/1
  q/1 -> Saturation/1
  Dot Product/1 -> 1/R/1
  1/R/1 -> Gain2/1
  Saturation/1 -> Dot Product/2, Dot Product1/2
  Dot Product1/1 -> iin/1

== system PowerFlowLib/Energy & Power Systems/Electrical/Converters/rectifier ==
  vqd0 : Inport
  cont : Inport  Port=2
  Vout : Inport  Port=3
  1/L : Gain  Gain=1/L  SaturateOnIntegerOverflow=on  OutDataTypeStr=Inherit: Same as input  ParamDataTypeStr=Inherit: Same as input
  Add : Sum  Inputs=+
  Demux : Demux  Outputs=3
  Mux : Mux  Inputs=3
  Product{,1..3} (4 alike) : Product  RndMeth=Zero
  Sqrt : Sqrt  SaturateOnIntegerOverflow=on
  Sum : Sum  Inputs=|+-
  Trigonometric Function : Trigonometry
  Trigonometric Function1 : Trigonometry  Operator=cos
  Trigonometric Function2 : Trigonometry  Operator=atan2
  iLstate : Integrator  LimitOutput=on  LowerSaturationLimit=0
  i_out : Outport
  iqd0 : Outport  Port=2
  wires:
  Vout/1 -> Sum/2
  vqd0/1 -> Demux/1, Product/1, Product/2
  Product/1 -> Add/1
  Add/1 -> Sqrt/1
  Sqrt/1 -> Product1/2
  cont/1 -> Product1/1
  Product1/1 -> Sum/1
  Trigonometric Function2/1 -> Trigonometric Function/1, Trigonometric Function1/1
  Trigonometric Function/1 -> Product2/1
  Trigonometric Function1/1 -> Product3/1
  Product2/1 -> Mux/1
  Product3/1 -> Mux/2
  Mux/1 -> iqd0/1
  Sum/1 -> 1/L/1
  1/L/1 -> iLstate/1
  iLstate/1 -> Product3/2, Product2/2, i_out/1
  Demux/1 -> Trigonometric Function2/1
  Demux/2 -> Trigonometric Function2/2

== system PowerFlowLib/Energy & Power Systems/Electrical/Coordinate Transformation/abc to qd0 ==
  note: abc to qd0 reference frame transform (using
      | Krause's notation q = direct axis, d = quadrature axis)
  V_a : Inport
  V_b : Inport  Port=2
  V_c : Inport  Port=3
  Fcn : Fcn  Expr=2/3*(u[1]*cos(0)+u[2]*cos(-2*pi/3)+u[3]*cos(2*pi/3))
  Fcn1 : Fcn  Expr=2/3*(u[1]*sin(0)+u[2]*sin(-2*pi/3)+u[3]*sin(2*pi/3))
  Fcn2 : Fcn  Expr=1/3*(u[1]+u[2]+u[3])
  Mux : Mux  Inputs=3
  V_q : Outport  InitialOutput=0
  V_d : Outport  Port=2  InitialOutput=0
  V_o : Outport  Port=3  InitialOutput=0
  wires:
  Fcn/1 -> V_q/1
  Fcn1/1 -> V_d/1
  Mux/1 -> Fcn/1, Fcn1/1, Fcn2/1
  V_c/1 -> Mux/3
  V_b/1 -> Mux/2
  V_a/1 -> Mux/1
  Fcn2/1 -> V_o/1

== system PowerFlowLib/Energy & Power Systems/Electrical/Coordinate Transformation/qd0 to abc ==
  note: qd0 to abc transformation (q = direct axis, d = quadrature axis)
  f_q : Inport
  f_d : Inport  Port=2
  f_o : Inport  Port=3
  Fcn : Fcn  Expr=u[1]*cos(0)+u[2]*sin(0)+u[3]
  Fcn1 : Fcn  Expr=u[1]*cos(-2*pi/3)+u[2]*sin(-2*pi/3)+u[3]
  Fcn2 : Fcn  Expr=u[1]*cos(2*pi/3)+u[2]*sin(2*pi/3)+u[3]
  Mux : Mux  Inputs=3
  f_a : Outport  InitialOutput=0
  f_b : Outport  Port=2  InitialOutput=0
  f_c : Outport  Port=3  InitialOutput=0
  wires:
  Fcn/1 -> f_a/1
  Fcn1/1 -> f_b/1
  Mux/1 -> Fcn/1, Fcn1/1, Fcn2/1
  f_o/1 -> Mux/3
  f_d/1 -> Mux/2
  f_q/1 -> Mux/1
  Fcn2/1 -> f_c/1

== system PowerFlowLib/Energy & Power Systems/Electrical/Coordinate Transformation/qde to qds ==
  note: Transform from synchronous (w = w_e) reference frame to stationary (w = 0) reference frame
  f_qe : Inport
  f_de : Inport  Port=2
  theta_e : Inport  Port=3
  Fcn : Fcn  Expr=u[1]*cos(u[3])+u[2]*sin(u[3])
  Fcn1 : Fcn  Expr=-u[1]*sin(u[3])+u[2]*cos(u[3])
  Mux : Mux  Inputs=3
  fq_s : Outport  InitialOutput=0
  fd_s : Outport  Port=2  InitialOutput=0
  wires:
  theta_e/1 -> Mux/3
  Fcn/1 -> fq_s/1
  Fcn1/1 -> fd_s/1
  Mux/1 -> Fcn1/1, Fcn/1
  f_de/1 -> Mux/2
  f_qe/1 -> Mux/1

== system PowerFlowLib/Energy & Power Systems/Electrical/Inverters/ inverter ==
  qqd0 : Inport
  VDC : Inport  Port=2
  iqd0 : Inport  Port=3
  Add : Sum  Inputs=+
  Product : Product  SaturateOnIntegerOverflow=on  InputSameDT=on  OutDataTypeStr=Inherit: Same as first input
  Product1 : Product  SaturateOnIntegerOverflow=on  InputSameDT=on  OutDataTypeStr=Inherit: Same as first input
  Product2 : Product  RndMeth=Zero
  Sqrt : Sqrt  SaturateOnIntegerOverflow=on
  Sum1 : Sum  Inputs=+
  Three-Phase Full Bridge Inverter CONSTANT FREQUENCY1 : Subsystem  mask{Tr=Trise, Tf=Tfall, Fsw=fsw, VCEsat=Vcesat, Nsw=Nofsw}
      mask prompts: Tr "Rise time for switching (s)"; Tf "Fall time for switching (s)"; Fsw "PWM Frequency (Hz)"; VCEsat "VCE saturation volt (V)"; Nsw "No. switches in inverter"
  Vqd0 : Outport
  Idc : Outport  Port=2
  Ploss : Outport  Port=3
  wires:
  Three-Phase Full Bridge Inverter CONSTANT FREQUENCY1/1(Total Loss) -> Ploss/1
  Sqrt/1 -> Three-Phase Full Bridge Inverter CONSTANT FREQUENCY1/2(Inverter current)
  Product2/1 -> Add/1
  Add/1 -> Sqrt/1
  [VDC] -> Three-Phase Full Bridge Inverter CONSTANT FREQUENCY1/1(Vdc)
  Sum1/1 -> Idc/1
  Product1/1 -> Sum1/1
  [qabc] -> Product1/2
  [qabc] -> Product/1
  qqd0/1 -> [qabc]
  iqd0/1 -> Product2/1, Product2/2, Product1/1
  Product/1 -> Vqd0/1
  VDC/1 -> [VDC]
  [VDC] -> Product/2

== system PowerFlowLib/Energy & Power Systems/Electrical/Inverters/1phs Inverter (2-level) - average ==
  m(t) : Inport
  vdc : Inport  Port=2
  iload : Inport  Port=3
  Constant : Constant
  Dot Product : Subsystem  mask(Dot Product){}
      mask help:
      | Inner (dot) product.
      | y = sum(conj(u1).*u2). The operand u1 corresponds to the top (or left) input port.
      mask init:
      | t=(0:.1:2*pi)';
      | x=cos(t);
      | y=sin(t);
      | r=0.05;
      mask Help: Computes the inner (dot) product of the inputs: sum(u1.*u2).  The inputs are vectors of the same length. Output is a scalar.
      mask Display: patch([x*r+0.5],[y*r+0.5])
  Dot Product1 : Subsystem  mask(Dot Product){}
      mask help:
      | Inner (dot) product.
      | y = sum(conj(u1).*u2). The operand u1 corresponds to the top (or left) input port.
      mask init:
      | t=(0:.1:2*pi)';
      | x=cos(t);
      | y=sin(t);
      | r=0.05;
      mask Help: Computes the inner (dot) product of the inputs: sum(u1.*u2).  The inputs are vectors of the same length. Output is a scalar.
      mask Display: patch([x*r+0.5],[y*r+0.5])
  Gain1 : Gain  Gain=2  SaturateOnIntegerOverflow=on  OutDataTypeStr=Inherit: Same as input  ParamDataTypeStr=Inherit: Same as input
  Sum : Sum  Inputs=+-  SaturateOnIntegerOverflow=on  InputSameDT=on  OutDataTypeStr=Inherit: Same as first input
  vout : Outport
  iin : Outport  Port=2
  wires:
  Dot Product1/1(Out1) -> iin/1
  Dot Product/1(Out1) -> vout/1
  iload/1 -> Dot Product1/2(In2)
  Sum/1 -> Dot Product1/1(In1), Dot Product/1(In1)
  vdc/1 -> Dot Product/2(In2)
  Constant/1 -> Sum/2
  m(t)/1 -> Gain1/1
  Gain1/1 -> Sum/1

== system PowerFlowLib/Energy & Power Systems/Electrical/Inverters/1phs Inverter (2-level) - switching ==
  m(t) : Inport
  vdc : Inport  Port=2
  iload : Inport  Port=3
  2-level PWM : Subsystem  mask(Two-level PWM block.){f_s=f_s}
      mask prompts: f_s "Switching frequency (Hz):"
      mask help: Two-level PWM block. PWM waveforms constructed by triangle comparison. Switching frequency adjustable. Duty ratio input is between 0 and 1. q1(t) is the switching function for switch 1, and q2(t) is the switching function for switch 2.
  Dot Product : Subsystem  mask(Dot Product){}
      mask help:
      | Inner (dot) product.
      | y = sum(conj(u1).*u2). The operand u1 corresponds to the top (or left) input port.
      mask init:
      | t=(0:.1:2*pi)';
      | x=cos(t);
      | y=sin(t);
      | r=0.05;
      mask Help: Computes the inner (dot) product of the inputs: sum(u1.*u2).  The inputs are vectors of the same length. Output is a scalar.
      mask Display: patch([x*r+0.5],[y*r+0.5])
  Dot Product1 : Subsystem  mask(Dot Product){}
      mask help:
      | Inner (dot) product.
      | y = sum(conj(u1).*u2). The operand u1 corresponds to the top (or left) input port.
      mask init:
      | t=(0:.1:2*pi)';
      | x=cos(t);
      | y=sin(t);
      | r=0.05;
      mask Help: Computes the inner (dot) product of the inputs: sum(u1.*u2).  The inputs are vectors of the same length. Output is a scalar.
      mask Display: patch([x*r+0.5],[y*r+0.5])
  Sum : Sum  Inputs=+-  SaturateOnIntegerOverflow=on  InputSameDT=on  OutDataTypeStr=Inherit: Same as first input
  vout : Outport
  iin : Outport  Port=2
  wires:
  m(t)/1 -> 2-level PWM/1(d(t))
  2-level PWM/1(q1(t)) -> Sum/1
  2-level PWM/2(q2(t)) -> Sum/2
  vdc/1 -> Dot Product/2(In2)
  Sum/1 -> Dot Product/1(In1), Dot Product1/1(In1)
  iload/1 -> Dot Product1/2(In2)
  Dot Product/1(Out1) -> vout/1
  Dot Product1/1(Out1) -> iin/1

== system PowerFlowLib/Energy & Power Systems/Electrical/Inverters/Current controller ==
  ia* : Inport
  ib* : Inport  Port=2
  ic* : Inport  Port=3
  ia : Inport  Port=4
  ib : Inport  Port=5
  ic : Inport  Port=6
  V_bus : Inport  Port=7
  1/2 : Gain  Gain=1/2  SaturateOnIntegerOverflow=on  OutDataTypeStr=Inherit: Same as input  ParamDataTypeStr=Inherit: Same as input
  CR_gain : Gain  Gain=CR_gain  SaturateOnIntegerOverflow=on  OutDataTypeStr=Inherit: Same as input  ParamDataTypeStr=Inherit: Same as input
  CR_gain_ : Gain  Gain=CR_gain  SaturateOnIntegerOverflow=on  OutDataTypeStr=Inherit: Same as input  ParamDataTypeStr=Inherit: Same as input
  CR_gain__ : Gain  Gain=CR_gain  SaturateOnIntegerOverflow=on  OutDataTypeStr=Inherit: Same as input  ParamDataTypeStr=Inherit: Same as input
  Constant : Constant  Value=V_IGBT
  Mux : Mux  Inputs=2
  Mux1 : Mux  Inputs=2
  Mux2 : Mux  Inputs=2
  R_IGBT : Gain  Gain=R_IGBT  SaturateOnIntegerOverflow=on  OutDataTypeStr=Inherit: Same as input  ParamDataTypeStr=Inherit: Same as input
  R_IGBT_ : Gain  Gain=R_IGBT  SaturateOnIntegerOverflow=on  OutDataTypeStr=Inherit: Same as input  ParamDataTypeStr=Inherit: Same as input
  R_IGBT__ : Gain  Gain=R_IGBT  SaturateOnIntegerOverflow=on  OutDataTypeStr=Inherit: Same as input  ParamDataTypeStr=Inherit: Same as input
  Sum{,1..5} (6 alike) : Sum  Inputs=+-  SaturateOnIntegerOverflow=on  InputSameDT=on  OutDataTypeStr=Inherit: Same as first input
  Sum6 : Sum  Inputs=-+  SaturateOnIntegerOverflow=on  InputSameDT=on  OutDataTypeStr=Inherit: Same as first input
  V_limit_b : Fcn  Expr=((u[2]>u[1])-(u[2]<(-u[1])))*u[1]+(u[2]<=u[1])*(u[2]>(-u[1]))*u[2]
  V_limit_c : Fcn  Expr=((u[2]>u[1])-(u[2]<(-u[1])))*u[1]+(u[2]<=u[1])*(u[2]>(-u[1]))*u[2]
  v_limit_a : Fcn  Expr=((u[2]>u[1])-(u[2]<(-u[1])))*u[1]+(u[2]<=u[1])*(u[2]>(-u[1]))*u[2]
  va : Outport
  vb : Outport  Port=2
  vc : Outport  Port=3
  wires:
  ia*/1 -> Sum/1
  Sum3/1 -> va/1
  Sum6/1 -> Mux2/1, Mux1/1, Mux/1
  Constant/1 -> Sum6/1
  1/2/1 -> Sum6/2
  R_IGBT__/1 -> Sum5/2
  R_IGBT_/1 -> Sum4/2
  R_IGBT/1 -> Sum3/2
  V_limit_c/1 -> Sum5/1
  V_limit_b/1 -> Sum4/1
  v_limit_a/1 -> Sum3/1
  ic/1 -> R_IGBT__/1, Sum2/2
  ib/1 -> R_IGBT_/1, Sum1/2
  ia/1 -> R_IGBT/1, Sum/2
  V_bus/1 -> 1/2/1
  ic*/1 -> Sum2/1
  ib*/1 -> Sum1/1
  Sum/1 -> CR_gain/1
  Sum1/1 -> CR_gain_/1
  Sum2/1 -> CR_gain__/1
  Mux2/1 -> V_limit_c/1
  Mux1/1 -> V_limit_b/1
  Mux/1 -> v_limit_a/1
  CR_gain__/1 -> Mux2/2
  CR_gain_/1 -> Mux1/2
  CR_gain/1 -> Mux/2
  Sum4/1 -> vb/1
  Sum5/1 -> vc/1

== system PowerFlowLib/Energy & Power Systems/Electrical/Inverters/Inverter (Average) ==
  Vdc : Inport
  ma : Inport  Port=2
  No. of battery cells1 : Gain  Gain=2
  No. of battery cells4 : Gain  Gain=0.5
  Product1 : Product  Inputs=3  RndMeth=Zero
  Product2 : Product  Inputs=*/  RndMeth=Zero
  Repeating Sequence : simulink/Sources/Repeating Sequence  rep_seq_t=[0 1/Freq]  rep_seq_y=[0 2*pi]
  abc 2 dq : Subsystem
  Vabc : Outport
  Vdq : Outport  Port=2
  mod index : Outport  Port=3
  wires:
  Vdc/1 -> No. of battery cells4/1
  No. of battery cells4/1 -> Product1/1
  ma/1 -> Product1/2
  [threevec] -> Product1/3
  Product1/1 -> abc 2 dq/1(I/P 3 phase), Vabc/1
  Repeating Sequence/1 -> abc 2 dq/2(angle)
  abc 2 dq/1("O/P 2 phase ") -> Vdq/1
  [vcmd] -> No. of battery cells1/1
  No. of battery cells1/1 -> Product2/1
  [Bus_vol] -> Product2/2
  Product2/1 -> mod index/1

== system PowerFlowLib/Energy & Power Systems/Electrical/Inverters/Inverter (Switching  Model) - Current  Control ==
  ia : Inport
  ib : Inport  Port=2
  ic : Inport  Port=3
  iaref : Inport  Port=4
  ibref : Inport  Port=5
  icref : Inport  Port=6
  Demux : Demux  Outputs=3
  Demux1 : Demux  Outputs=3
  Integrator : Integrator
  Mux : Mux  Inputs=3
  Product : Product  RndMeth=Zero
  Product1 : Product  Inputs=*/  RndMeth=Zero
  Product2 : Product  Inputs=*/  RndMeth=Zero
  Relay : Relay  OnSwitchValue=1  OffSwitchValue=-1  OnOutputValue=-1  OffOutputValue=1
  Sum{,1..3} (4 alike) : Sum  Inputs=|+-
  Va : Outport
  Vb : Outport  Port=2
  Vc : Outport  Port=3
  iat : Outport  Port=4
  ibt : Outport  Port=5
  ict : Outport  Port=6
  wires:
  [Back_emf] -> Sum3/2
  Sum3/1 -> Demux1/1, Integrator/1
  Product/1 -> Sum3/1
  Product2/1 -> Relay/1
  [Hys_band] -> Product2/2
  Mux/1 -> Product2/1
  Relay/1 -> Product/1
  Demux1/1 -> Va/1
  Demux1/3 -> Vc/1
  Demux1/2 -> Vb/1
  Demux/3 -> ict/1
  Demux/2 -> ibt/1
  Demux/1 -> iat/1
  Product1/1 -> Demux/1
  [Lls] -> Product1/2
  Integrator/1 -> Product1/1
  [Bus_vol] -> Product/2
  Sum/1 -> Mux/1
  Sum2/1 -> Mux/3
  icref/1 -> Sum2/2
  ic/1 -> Sum2/1
  Sum1/1 -> Mux/2
  ibref/1 -> Sum1/2
  ib/1 -> Sum1/1
  iaref/1 -> Sum/2
  ia/1 -> Sum/1

== system PowerFlowLib/Energy & Power Systems/Electrical/Inverters/three-phase  full-bridge  inverter ==
  qa : Inport
  qb : Inport  Port=2
  qc : Inport  Port=3
  VDC : Inport  Port=4
  ia : Inport  Port=5
  ib : Inport  Port=6
  ic : Inport  Port=7
  Data Type Conversion : DataTypeConversion  SaturateOnIntegerOverflow=on  RndMeth=Zero
  Data Type Conversion1 : DataTypeConversion  SaturateOnIntegerOverflow=on  RndMeth=Zero
  Data Type Conversion2 : DataTypeConversion  SaturateOnIntegerOverflow=on  RndMeth=Zero
  Product{,1..5} (6 alike) : Product  SaturateOnIntegerOverflow=on  InputSameDT=on  OutDataTypeStr=Inherit: Same as first input
  Sum : Sum  Inputs=|+++  SaturateOnIntegerOverflow=on  InputSameDT=on  OutDataTypeStr=Inherit: Same as first input
  Sum4 : Sum  Inputs=|+-  SaturateOnIntegerOverflow=on  InputSameDT=on  OutDataTypeStr=Inherit: Same as first input
  Sum5 : Sum  Inputs=|+-  SaturateOnIntegerOverflow=on  InputSameDT=on  OutDataTypeStr=Inherit: Same as first input
  Sum6 : Sum  Inputs=|+-  SaturateOnIntegerOverflow=on  InputSameDT=on  OutDataTypeStr=Inherit: Same as first input
  Idc : Outport
  Vab : Outport  Port=2
  Vbc : Outport  Port=3
  Vca : Outport  Port=4
  wires:
  [VAN] -> Sum6/2
  [VCN] -> Sum6/1
  Product1/1 -> [VBN]
  Product2/1 -> [VCN]
  Product/1 -> [VAN]
  Sum6/1 -> Vca/1
  Sum5/1 -> [vbc], Vbc/1
  [VCN] -> Sum5/2
  [VBN] -> Sum5/1
  Sum4/1 -> [vab], Vab/1
  [VBN] -> Sum4/2
  [VAN] -> Sum4/1
  Sum/1 -> Idc/1
  Product5/1 -> Sum/3
  ic/1 -> Product5/2
  Product4/1 -> Sum/2
  ib/1 -> Product4/2
  Product3/1 -> Sum/1
  ia/1 -> Product3/2
  [VDC] -> Product2/2
  qc/1 -> Data Type Conversion2/1
  [VDC] -> Product1/2
  qb/1 -> Data Type Conversion1/1
  [VDC] -> Product/2
  VDC/1 -> [VDC]
  qa/1 -> Data Type Conversion/1
  Data Type Conversion/1 -> Product3/1, Product/1
  Data Type Conversion1/1 -> Product4/1, Product1/1
  Data Type Conversion2/1 -> Product5/1, Product2/1

== system PowerFlowLib/Energy & Power Systems/Electrical/Inverters/three-phase  full-bridge  inverter1 ==
  qabc : Inport
  VDC : Inport  Port=2
  iabc : Inport  Port=3
  Product : Product  SaturateOnIntegerOverflow=on  InputSameDT=on  OutDataTypeStr=Inherit: Same as first input
  Product1 : Product  SaturateOnIntegerOverflow=on  InputSameDT=on  OutDataTypeStr=Inherit: Same as first input
  Sum1 : Sum  Inputs=+
  Vabc : Outport
  Idc : Outport  Port=2
  wires:
  [VDC] -> Product/2
  VDC/1 -> [VDC]
  Product/1 -> Vabc/1
  iabc/1 -> Product1/1
  qabc/1 -> [qabc]
  [qabc] -> Product/1
  [qabc] -> Product1/2
  Product1/1 -> Sum1/1
  Sum1/1 -> Idc/1

== system PowerFlowLib/Energy & Power Systems/Electrical/Loads/Constant Current Load ==
  I_rms : Inport
  P.F. : Inport  Port=2
  Vabc : Inport  Port=3
  Eta1 : Inport  Port=4
  Constant : Constant  Value=[0 -2*pi/3 2*pi/3]
  Demux : Demux  Outputs=3
  Fcn1 : Fcn  Expr=(u(1)<=1)*(1-u(1))
  Math Function : Math  Operator=square  SaturateOnIntegerOverflow=on
  Mean Value : powerlib_extras/Measurements/Mean Value  Period=1/60
  Product{,1..6} (7 alike) : Product  RndMeth=Zero
  Sqrt : Sqrt  SaturateOnIntegerOverflow=on
  Sum : Sum  Inputs=|+-
  Sum1 : Sum
  Trigonometric Function : Trigonometry  Operator=acos
  Trigonometric Function1 : Trigonometry
  Trigonometric Function2 : Trigonometry  Operator=atan2
  Trigonometric Function3 : Trigonometry  Operator=cos
  Trigonometric Function4 : Trigonometry
  abc to qd0 : Subsystem
  iabc : Outport
  P : Outport  Port=2
  P_loss1 : Outport  Port=3
  Q : Outport  Port=4
  wires:
  Math Function/1 -> Mean Value/1
  Mean Value/1 -> Sqrt/1
  Sqrt/1 -> Product4/2, Product6/2  "RMS"
  I_rms/1 -> Product/1, Product1/1
  P.F./1 -> Product/2, Trigonometric Function/1
  Trigonometric Function/1 -> Trigonometric Function1/1
  Trigonometric Function1/1 -> Product1/2
  Product/1 -> Product2/1, Product6/1
  Vabc/1 -> Demux/1
  Demux/1 -> abc to qd0/1(V_a), Math Function/1
  Demux/2 -> abc to qd0/2(V_b)
  Demux/3 -> abc to qd0/3(V_c)
  Trigonometric Function3/1 -> Product2/2
  Trigonometric Function4/1 -> Product3/2
  Trigonometric Function2/1 -> Sum/1
  Constant/1 -> Sum/2
  Sum/1 -> Trigonometric Function3/1, Trigonometric Function4/1
  Product2/1 -> Sum1/1
  Product3/1 -> Sum1/2
  Sum1/1 -> iabc/1
  abc to qd0/2(V_d) -> Trigonometric Function2/1
  abc to qd0/1(V_q) -> Trigonometric Function2/2
  Product1/1 -> Product3/1, Product4/1
  Eta1/1 -> Fcn1/1
  Product5/1 -> P_loss1/1
  Product6/1 -> P/1, Product5/1
  Product4/1 -> Q/1
  Fcn1/1 -> Product5/2
